simulink model "P702_NI_SoftECU"  (R2019a)
settings: Solver=ode1  StartTime=0.0  StopTime=Inf  FixedStep=0.001  RelTol=1e-3  EnableMultiTasking=on
PreLoadFcn:
  | run '.\VeriStand_BlockSet\NIVeriStandAddPaths.m'
undefined symbols (not defined in the file or in its folder): magnitude
libraries: simulink x83, simulink_extras x1
(part 66 of 76)

== system P702_NI_SoftECU/Output/Subsystem1/To_NI_HIL/Soft_ABS/ABS_BrkBst_Data ==
  in_port : Inport
  BrkTotTqRqDrv_No_Cnt : Terminator
  BrkTotTqRqDrv_No_Cs : Terminator
  BrkTot_Tq_RqDrv : Terminator
  bus_selector : BusSelector  OutputSignals=BrkTot_Tq_RqDrv,BrkTotTqRqDrv_No_Cs,BrkTotTqRqDrv_No_Cnt
  wires:
  in_port/1 -> bus_selector/1  "Subsystem1"
  bus_selector/1 -> BrkTot_Tq_RqDrv/1  "<BrkTot_Tq_RqDrv>"
  bus_selector/2 -> BrkTotTqRqDrv_No_Cs/1  "<BrkTotTqRqDrv_No_Cs>"
  bus_selector/3 -> BrkTotTqRqDrv_No_Cnt/1  "<BrkTotTqRqDrv_No_Cnt>"

== system P702_NI_SoftECU/Output/Subsystem1/To_NI_HIL/Soft_ABS/Accel_Data ==
  in_port : Inport
  VehLat2_A_Actl : Terminator
  VehLong2_A_Actl : Terminator
  bus_selector : BusSelector  OutputSignals=VehLong2_A_Actl,VehLat2_A_Actl
  wires:
  in_port/1 -> bus_selector/1  "Subsystem1"
  bus_selector/1 -> VehLong2_A_Actl/1  "<VehLong2_A_Actl>"
  bus_selector/2 -> VehLat2_A_Actl/1  "<VehLat2_A_Actl>"

== system P702_NI_SoftECU/Output/Subsystem1/To_NI_HIL/Soft_ABS/BrakeSnData_3 ==
  in_port : Inport
  VehLatComp_A_Actl : Terminator
  VehLongComp_A_Actl : Terminator
  VehOverGnd_V_Est : Terminator
  VehYawComp_W_Actl : Terminator
  bus_selector : BusSelector  OutputSignals=VehYawComp_W_Actl,VehOverGnd_V_Est,VehLongComp_A_Actl,VehLatComp_A_Actl
  wires:
  in_port/1 -> bus_selector/1  "Subsystem1"
  bus_selector/1 -> VehYawComp_W_Actl/1  "<VehYawComp_W_Actl>"
  bus_selector/2 -> VehOverGnd_V_Est/1  "<VehOverGnd_V_Est>"
  bus_selector/3 -> VehLongComp_A_Actl/1  "<VehLongComp_A_Actl>"
  bus_selector/4 -> VehLatComp_A_Actl/1  "<VehLatComp_A_Actl>"

== system P702_NI_SoftECU/Output/Subsystem1/To_NI_HIL/Soft_ABS/BrakeSnData_4 ==
  in_port : Inport
  BrkTot_Tq_Actl : Terminator
  VehRolComp_W_Actl : Terminator
  VehVertComp_A_Actl : Terminator
  bus_selector : BusSelector  OutputSignals=VehVertComp_A_Actl,VehRolComp_W_Actl,BrkTot_Tq_Actl
  wires:
  in_port/1 -> bus_selector/1  "Subsystem1"
  bus_selector/1 -> VehVertComp_A_Actl/1  "<VehVertComp_A_Actl>"
  bus_selector/2 -> VehRolComp_W_Actl/1  "<VehRolComp_W_Actl>"
  bus_selector/3 -> BrkTot_Tq_Actl/1  "<BrkTot_Tq_Actl>"

== system P702_NI_SoftECU/Output/Subsystem1/To_NI_HIL/Soft_ABS/BrakeSnData_5 ==
  in_port : Inport
  SteWhlComp_An_Est : Terminator
  bus_selector : BusSelector  OutputSignals=SteWhlComp_An_Est
  wires:
  in_port/1 -> bus_selector/1  "Subsystem1"
  bus_selector/1 -> SteWhlComp_An_Est/1  "<SteWhlComp_An_Est>"

== system P702_NI_SoftECU/Output/Subsystem1/To_NI_HIL/Soft_ABS/BrakeSysFeatures ==
  in_port : Inport
  VehVActlBrk_No_Cnt : Terminator
  VehVActlBrk_No_Cs : Terminator
  Veh_V_ActlBrk : Terminator
  bus_selector : BusSelector  OutputSignals=Veh_V_ActlBrk,VehVActlBrk_No_Cs,VehVActlBrk_No_Cnt
  wires:
  in_port/1 -> bus_selector/1  "Subsystem1"
  bus_selector/1 -> Veh_V_ActlBrk/1  "<Veh_V_ActlBrk>"
  bus_selector/2 -> VehVActlBrk_No_Cs/1  "<VehVActlBrk_No_Cs>"
  bus_selector/3 -> VehVActlBrk_No_Cnt/1  "<VehVActlBrk_No_Cnt>"

== system P702_NI_SoftECU/Output/Subsystem1/To_NI_HIL/Soft_ABS/BrakeSysFeatures_2 ==
  in_port : Inport
  BpedMove_D_Actl : Terminator
  BpedMove_No_Cnt : Terminator
  BpedMove_No_Cs : Terminator
  bus_selector : BusSelector  OutputSignals=BpedMove_D_Actl,BpedMove_No_Cs,BpedMove_No_Cnt
  wires:
  in_port/1 -> bus_selector/1  "Subsystem1"
  bus_selector/1 -> BpedMove_D_Actl/1  "<BpedMove_D_Actl>"
  bus_selector/2 -> BpedMove_No_Cs/1  "<BpedMove_No_Cs>"
  bus_selector/3 -> BpedMove_No_Cnt/1  "<BpedMove_No_Cnt>"

== system P702_NI_SoftECU/Output/Subsystem1/To_NI_HIL/Soft_ABS/DesiredTorqBrk ==
  in_port : Inport
  AccBrkActv_B_Actl : Terminator
  AccBrkPrchgActv_B_Actl : Terminator
  AccBrkTotTqMn_B_Actl : Terminator
  AccStopActv_B_ActlBrk : Terminator
  CmbbBaSensInc_B_Actl : Terminator
  CmbbBrkDecel_B_Actl : Terminator
  CmbbBrkPrchg_B_Actl : Terminator
  VehLongOvrGnd_A_Est : Terminator
  VehStop_D_Stat : Terminator
  VehicleStationary : Terminator
  bus_selector : BusSelector  OutputSignals=AccBrkPrchgActv_B_Actl,AccBrkActv_B_Actl,AccStopActv_B_ActlBrk,CmbbBrkPrchg_B_Actl,CmbbBaSensInc_B_Actl,CmbbBrkDecel_B_Actl,VehicleStationary,VehStop_D_Stat,VehLongOvrGnd_A_Est,AccBrkTotTqMn_B_Actl
  wires:
  in_port/1 -> bus_selector/1  "Subsystem1"
  bus_selector/1 -> AccBrkPrchgActv_B_Actl/1  "<AccBrkPrchgActv_B_Actl>"
  bus_selector/2 -> AccBrkActv_B_Actl/1  "<AccBrkActv_B_Actl>"
  bus_selector/3 -> AccStopActv_B_ActlBrk/1  "<AccStopActv_B_ActlBrk>"
  bus_selector/4 -> CmbbBrkPrchg_B_Actl/1  "<CmbbBrkPrchg_B_Actl>"
  bus_selector/5 -> CmbbBaSensInc_B_Actl/1  "<CmbbBaSensInc_B_Actl>"
  bus_selector/6 -> CmbbBrkDecel_B_Actl/1  "<CmbbBrkDecel_B_Actl>"
  bus_selector/7 -> VehicleStationary/1  "<VehicleStationary>"
  bus_selector/8 -> VehStop_D_Stat/1  "<VehStop_D_Stat>"
  bus_selector/9 -> VehLongOvrGnd_A_Est/1  "<VehLongOvrGnd_A_Est>"
  bus_selector/10 -> AccBrkTotTqMn_B_Actl/1  "<AccBrkTotTqMn_B_Actl>"

== system P702_NI_SoftECU/Output/Subsystem1/To_NI_HIL/Soft_ABS/ToCarSim ==
  in_port : Inport
  MCPressure : Terminator
  bus_selector : BusSelector  OutputSignals=MCPressure
  wires:
  in_port/1 -> bus_selector/1  "Subsystem1"
  bus_selector/1 -> MCPressure/1  "<MCPressure>"

== system P702_NI_SoftECU/Output/Subsystem1/To_NI_HIL/Soft_ABS/WheelData ==
  in_port : Inport
  WhlDirRl_D_Actl : Terminator
  WhlDirRr_D_Actl : Terminator
  bus_selector : BusSelector  OutputSignals=WhlDirRl_D_Actl,WhlDirRr_D_Actl
  wires:
  in_port/1 -> bus_selector/1  "Subsystem1"
  bus_selector/1 -> WhlDirRl_D_Actl/1  "<WhlDirRl_D_Actl>"
  bus_selector/2 -> WhlDirRr_D_Actl/1  "<WhlDirRr_D_Actl>"

== system P702_NI_SoftECU/Output/Subsystem1/To_NI_HIL/Soft_ABS/WheelSpeed ==
  in_port : Inport
  WhlFl_W_Meas : Terminator
  WhlFr_W_Meas : Terminator
  WhlRl_W_Meas : Terminator
  WhlRotatFl_No_Cnt : Terminator
  WhlRotatFr_No_Cnt : Terminator
  WhlRotatRl_No_Cnt : Terminator
  WhlRotatRr_No_Cnt : Terminator
  WhlRr_W_Meas : Terminator
  bus_selector : BusSelector  OutputSignals=WhlFl_W_Meas,WhlFr_W_Meas,WhlRl_W_Meas,WhlRr_W_Meas,WhlRotatFl_No_Cnt,WhlRotatFr_No_Cnt,WhlRotatRl_No_Cnt,WhlRotatRr_No_Cnt
  wires:
  in_port/1 -> bus_selector/1  "Subsystem1"
  bus_selector/1 -> WhlFl_W_Meas/1  "<WhlFl_W_Meas>"
  bus_selector/2 -> WhlFr_W_Meas/1  "<WhlFr_W_Meas>"
  bus_selector/3 -> WhlRl_W_Meas/1  "<WhlRl_W_Meas>"
  bus_selector/4 -> WhlRr_W_Meas/1  "<WhlRr_W_Meas>"
  bus_selector/5 -> WhlRotatFl_No_Cnt/1  "<WhlRotatFl_No_Cnt>"
  bus_selector/6 -> WhlRotatFr_No_Cnt/1  "<WhlRotatFr_No_Cnt>"
  bus_selector/7 -> WhlRotatRl_No_Cnt/1  "<WhlRotatRl_No_Cnt>"
  bus_selector/8 -> WhlRotatRr_No_Cnt/1  "<WhlRotatRr_No_Cnt>"

== system P702_NI_SoftECU/Output/Subsystem1/To_NI_HIL/Soft_ABS/Yaw_Data ==
  in_port : Inport
  VehYaw_W_Actl : Terminator
  bus_selector : BusSelector  OutputSignals=VehYaw_W_Actl
  wires:
  in_port/1 -> bus_selector/1  "Subsystem1"
  bus_selector/1 -> VehYaw_W_Actl/1  "<VehYaw_W_Actl>"

== system P702_NI_SoftECU/Output/Subsystem1/To_NI_HIL/Soft_BCM/BodyInfo_3 ==
  in_port : Inport
  Ignition_Status : Terminator
  bus_selector : BusSelector  OutputSignals=Ignition_Status
  wires:
  in_port/1 -> bus_selector/1  "Subsystem1"
  bus_selector/1 -> Ignition_Status/1  "<Ignition_Status>"

== system P702_NI_SoftECU/Output/Subsystem1/To_NI_HIL/Soft_BCM/Cluster_Info1 ==
  in_port : Inport
  OdometerMasterValue : Terminator
  OdometerMasterValue_UB : Terminator
  bus_selector : BusSelector  OutputSignals=OdometerMasterValue,OdometerMasterValue_UB
  wires:
  in_port/1 -> bus_selector/1  "Subsystem1"
  bus_selector/1 -> OdometerMasterValue/1  "<OdometerMasterValue>"
  bus_selector/2 -> OdometerMasterValue_UB/1  "<OdometerMasterValue_UB>"

== system P702_NI_SoftECU/Output/Subsystem1/To_NI_HIL/Soft_BCM/GGCC_Config_Mgmt_ID ==
  in_port : Inport
  Byte_{0..7} (8 alike) : Terminator
  bus_selector : BusSelector  OutputSignals=Byte_0,Byte_1,Byte_2,Byte_3,Byte_4,Byte_5,Byte_6,Byte_7
  wires:
  in_port/1 -> bus_selector/1  "Subsystem1"
  bus_selector/1 -> Byte_0/1  "<Byte_0>"
  bus_selector/2 -> Byte_1/1  "<Byte_1>"
  bus_selector/3 -> Byte_2/1  "<Byte_2>"
  bus_selector/4 -> Byte_3/1  "<Byte_3>"
  bus_selector/5 -> Byte_4/1  "<Byte_4>"
  bus_selector/6 -> Byte_5/1  "<Byte_5>"
  bus_selector/7 -> Byte_6/1  "<Byte_6>"
  bus_selector/8 -> Byte_7/1  "<Byte_7>"

== system P702_NI_SoftECU/Output/Subsystem1/To_NI_HIL/Soft_BCM/Personality_BCM2_Data ==
  in_port : Inport
  RecallEvent_No_Cnt : Terminator
  bus_selector : BusSelector  OutputSignals=RecallEvent_No_Cnt
  wires:
  in_port/1 -> bus_selector/1  "Subsystem1"
  bus_selector/1 -> RecallEvent_No_Cnt/1  "<RecallEvent_No_Cnt>"

== system P702_NI_SoftECU/Output/Subsystem1/To_NI_HIL/Soft_ECM/EngBrakeData ==
  in_port : Inport
  ACCStopMde_D_Rq : Terminator
  Cc_Stat_D_Actl : Terminator
  CmbbEngTqMn_B_Rq : Terminator
  PrplTqMnSat_B_Actl : Terminator
  bus_selector : BusSelector  OutputSignals=CmbbEngTqMn_B_Rq,ACCStopMde_D_Rq,PrplTqMnSat_B_Actl,Cc_Stat_D_Actl
  wires:
  in_port/1 -> bus_selector/1  "Subsystem1"
  bus_selector/1 -> CmbbEngTqMn_B_Rq/1  "<CmbbEngTqMn_B_Rq>"
  bus_selector/2 -> ACCStopMde_D_Rq/1  "<ACCStopMde_D_Rq>"
  bus_selector/3 -> PrplTqMnSat_B_Actl/1  "<PrplTqMnSat_B_Actl>"
  bus_selector/4 -> Cc_Stat_D_Actl/1  "<Cc_Stat_D_Actl>"

== system P702_NI_SoftECU/Output/Subsystem1/To_NI_HIL/Soft_ECM/EngVehicleSpThrottle ==
  in_port : Inport
  EngAout_N_Actl : Terminator
  bus_selector : BusSelector  OutputSignals=EngAout_N_Actl
  wires:
  in_port/1 -> bus_selector/1  "Subsystem1"
  bus_selector/1 -> EngAout_N_Actl/1  "<EngAout_N_Actl>"

== system P702_NI_SoftECU/Output/Subsystem1/To_NI_HIL/Soft_ECM/EngVehicleSpThrottle2 ==
  in_port : Inport
  Veh_V_ActlEng : Terminator
  bus_selector : BusSelector  OutputSignals=Veh_V_ActlEng
  wires:
  in_port/1 -> bus_selector/1  "Subsystem1"
  bus_selector/1 -> Veh_V_ActlEng/1  "<Veh_V_ActlEng>"

== system P702_NI_SoftECU/Output/Subsystem1/To_NI_HIL/Soft_MRR/MRR_Detection ==
  in_port : Inport
  MRR_Detection_001 : Subsystem
  MRR_Detection_002 : Subsystem
  MRR_Detection_003 : Subsystem
  bus_selector : BusSelector  OutputSignals=MRR_Detection_001,MRR_Detection_002,MRR_Detection_003
  wires:
  in_port/1 -> bus_selector/1  "Subsystem1"
  bus_selector/1 -> MRR_Detection_001/1(in_port)  "<MRR_Detection_001>"
  bus_selector/2 -> MRR_Detection_002/1(in_port)  "<MRR_Detection_002>"
  bus_selector/3 -> MRR_Detection_003/1(in_port)  "<MRR_Detection_003>"

== system P702_NI_SoftECU/Output/Subsystem1/To_NI_HIL/Soft_PCM/EngBrakeData ==
  in_port : Inport
  BpedDrvAppl_D_Actl : Terminator
  BrkOnOffSwtch_D_Actl : Terminator
  bus_selector : BusSelector  OutputSignals=BrkOnOffSwtch_D_Actl,BpedDrvAppl_D_Actl
  wires:
  in_port/1 -> bus_selector/1  "Subsystem1"
  bus_selector/1 -> BrkOnOffSwtch_D_Actl/1  "<BrkOnOffSwtch_D_Actl>"
  bus_selector/2 -> BpedDrvAppl_D_Actl/1  "<BpedDrvAppl_D_Actl>"

== system P702_NI_SoftECU/Output/Subsystem1/To_NI_HIL/Soft_PCM/EngVehicleSpThottle2 ==
  in_port : Inport
  GearRvrse_D_Actl : Terminator
  Veh_V_ActlEng : Terminator
  Veh_V_RqCcSet : Terminator
  bus_selector : BusSelector  OutputSignals=Veh_V_ActlEng,GearRvrse_D_Actl,Veh_V_RqCcSet
  wires:
  in_port/1 -> bus_selector/1  "Subsystem1"
  bus_selector/1 -> Veh_V_ActlEng/1  "<Veh_V_ActlEng>"
  bus_selector/2 -> GearRvrse_D_Actl/1  "<GearRvrse_D_Actl>"
  bus_selector/3 -> Veh_V_RqCcSet/1  "<Veh_V_RqCcSet>"

== system P702_NI_SoftECU/Output/Subsystem1/To_NI_HIL/Soft_PCM/EngVehicleSpThrottle ==
  in_port : Inport
  ApedPosPcActl_No_Cs : Terminator
  ApedPos_PcRate_ActlArb : Terminator
  ApedPos_Pc_ActlArb : Terminator
  ApedPos_Pc_ActlArb_No_Cnt : Terminator
  EngAout_N_Actl : Terminator
  bus_selector : BusSelector  OutputSignals=EngAout_N_Actl,ApedPos_Pc_ActlArb,ApedPos_PcRate_ActlArb,ApedPosPcActl_No_Cs,ApedPos_Pc_ActlArb_No_Cnt
  wires:
  in_port/1 -> bus_selector/1  "Subsystem1"
  bus_selector/1 -> EngAout_N_Actl/1  "<EngAout_N_Actl>"
  bus_selector/2 -> ApedPos_Pc_ActlArb/1  "<ApedPos_Pc_ActlArb>"
  bus_selector/3 -> ApedPos_PcRate_ActlArb/1  "<ApedPos_PcRate_ActlArb>"
  bus_selector/4 -> ApedPosPcActl_No_Cs/1  "<ApedPosPcActl_No_Cs>"
  bus_selector/5 -> ApedPos_Pc_ActlArb_No_Cnt/1  "<ApedPos_Pc_ActlArb_No_Cnt>"

== system P702_NI_SoftECU/Output/Subsystem1/To_NI_HIL/Soft_PCM/EngineClimateData ==
  in_port : Inport
  AirAmb_Te_Actl : Terminator
  AirAmb_Te_ActlFilt : Terminator
  EngAout_Aa_Actl : Terminator
  bus_selector : BusSelector  OutputSignals=EngAout_Aa_Actl,AirAmb_Te_Actl,AirAmb_Te_ActlFilt
  wires:
  in_port/1 -> bus_selector/1  "Subsystem1"
  bus_selector/1 -> EngAout_Aa_Actl/1  "<EngAout_Aa_Actl>"
  bus_selector/2 -> AirAmb_Te_Actl/1  "<AirAmb_Te_Actl>"
  bus_selector/3 -> AirAmb_Te_ActlFilt/1  "<AirAmb_Te_ActlFilt>"

== system P702_NI_SoftECU/Output/Subsystem1/To_NI_HIL/Soft_PCM/EngineClutchData ==
  in_port : Inport
  CluPdlPosPcMeas_D_Qf : Terminator
  CluPdlPos_Pc_Meas : Terminator
  CluPdl_PcRate_Actl : Terminator
  bus_selector : BusSelector  OutputSignals=CluPdl_PcRate_Actl,CluPdlPos_Pc_Meas,CluPdlPosPcMeas_D_Qf
  wires:
  in_port/1 -> bus_selector/1  "Subsystem1"
  bus_selector/1 -> CluPdl_PcRate_Actl/1  "<CluPdl_PcRate_Actl>"
  bus_selector/2 -> CluPdlPos_Pc_Meas/1  "<CluPdlPos_Pc_Meas>"
  bus_selector/3 -> CluPdlPosPcMeas_D_Qf/1  "<CluPdlPosPcMeas_D_Qf>"

== system P702_NI_SoftECU/Output/Subsystem1/To_NI_HIL/Soft_PCM/EngineData_7 ==
  in_port : Inport
  FuelFlw_Vl_Dsply : Terminator
  OdoCount : Terminator
  bus_selector : BusSelector  OutputSignals=OdoCount,FuelFlw_Vl_Dsply
  wires:
  in_port/1 -> bus_selector/1  "Subsystem1"
  bus_selector/1 -> OdoCount/1  "<OdoCount>"
  bus_selector/2 -> FuelFlw_Vl_Dsply/1  "<FuelFlw_Vl_Dsply>"

== system P702_NI_SoftECU/Output/Subsystem1/To_NI_HIL/Soft_PCM/PowertrainData_10 ==
  in_port : Inport
  GearLvr_D_ActlDrv : Terminator
  GearPos_No_Cnt : Terminator
  GearPos_No_Cs : Terminator
  bus_selector : BusSelector  OutputSignals=GearPos_No_Cs,GearPos_No_Cnt,GearLvr_D_ActlDrv
  wires:
  in_port/1 -> bus_selector/1  "Subsystem1"
  bus_selector/1 -> GearPos_No_Cs/1  "<GearPos_No_Cs>"
  bus_selector/2 -> GearPos_No_Cnt/1  "<GearPos_No_Cnt>"
  bus_selector/3 -> GearLvr_D_ActlDrv/1  "<GearLvr_D_ActlDrv>"

== system P702_NI_SoftECU/Output/Subsystem1/To_NI_HIL/Soft_PCM/TorqueDataEngFlags ==
  in_port : Inport
  PrplWhlTotTqRq_No_Cs : Terminator
  PrplWhlTot_Tq_Rq : Terminator
  PrplWhlTot_Tq_Rq_No_Cnt : Terminator
  bus_selector : BusSelector  OutputSignals=PrplWhlTot_Tq_Rq,PrplWhlTotTqRq_No_Cs,PrplWhlTot_Tq_Rq_No_Cnt
  wires:
  in_port/1 -> bus_selector/1  "Subsystem1"
  bus_selector/1 -> PrplWhlTot_Tq_Rq/1  "<PrplWhlTot_Tq_Rq>"
  bus_selector/2 -> PrplWhlTotTqRq_No_Cs/1  "<PrplWhlTotTqRq_No_Cs>"
  bus_selector/3 -> PrplWhlTot_Tq_Rq_No_Cnt/1  "<PrplWhlTot_Tq_Rq_No_Cnt>"

== system P702_NI_SoftECU/Output/Subsystem1/To_NI_HIL/Soft_PCM/VehicleOperatingModes ==
  in_port : Inport
  ElPw_D_Stat : Terminator
  ElPw_D_StatStrtStop : Terminator
  Eng_D_Stat : Terminator
  PrplWhlTot2_Tq_Rq : Terminator
  PwPckTq_D_Stat : Terminator
  bus_selector : BusSelector  OutputSignals=Eng_D_Stat,PwPckTq_D_Stat,PrplWhlTot2_Tq_Rq,ElPw_D_StatStrtStop,ElPw_D_Stat
  wires:
  in_port/1 -> bus_selector/1  "Subsystem1"
  bus_selector/1 -> Eng_D_Stat/1  "<Eng_D_Stat>"
  bus_selector/2 -> PwPckTq_D_Stat/1  "<PwPckTq_D_Stat>"
  bus_selector/3 -> PrplWhlTot2_Tq_Rq/1  "<PrplWhlTot2_Tq_Rq>"
  bus_selector/4 -> ElPw_D_StatStrtStop/1  "<ElPw_D_StatStrtStop>"
  bus_selector/5 -> ElPw_D_Stat/1  "<ElPw_D_Stat>"

== system P702_NI_SoftECU/Output/Subsystem1/To_NI_HIL/Soft_RCM/Accel_Data ==
  in_port : Inport
  VehLat2_A_Actl : Terminator
  VehLatAActl_D_Qf : Terminator
  VehLatLongVert_No_Cnt : Terminator
  VehLatLongVert_No_Cs : Terminator
  VehLong2_A_Actl : Terminator
  VehLongAActl_D_Qf : Terminator
  VehVert2_A_Actl : Terminator
  VehVertAActl_D_Qf : Terminator
  bus_selector : BusSelector  OutputSignals=VehLat2_A_Actl,VehLong2_A_Actl,VehVert2_A_Actl,VehLatLongVert_No_Cnt,VehLatLongVert_No_Cs,VehLatAActl_D_Qf,VehLongAActl_D_Qf,VehVertAActl_D_Qf
  wires:
  in_port/1 -> bus_selector/1  "Subsystem1"
  bus_selector/1 -> VehLat2_A_Actl/1  "<VehLat2_A_Actl>"
  bus_selector/2 -> VehLong2_A_Actl/1  "<VehLong2_A_Actl>"
  bus_selector/3 -> VehVert2_A_Actl/1  "<VehVert2_A_Actl>"
  bus_selector/4 -> VehLatLongVert_No_Cnt/1  "<VehLatLongVert_No_Cnt>"
  bus_selector/5 -> VehLatLongVert_No_Cs/1  "<VehLatLongVert_No_Cs>"
  bus_selector/6 -> VehLatAActl_D_Qf/1  "<VehLatAActl_D_Qf>"
  bus_selector/7 -> VehLongAActl_D_Qf/1  "<VehLongAActl_D_Qf>"
  bus_selector/8 -> VehVertAActl_D_Qf/1  "<VehVertAActl_D_Qf>"

== system P702_NI_SoftECU/Output/Subsystem1/To_NI_HIL/Soft_RCM/RCMStatusMessage2 ==
  in_port : Inport
  FirstRowBuckleDriver : Terminator
  RstrnImpactEvntStatus : Terminator
  bus_selector : BusSelector  OutputSignals=RstrnImpactEvntStatus,FirstRowBuckleDriver
  wires:
  in_port/1 -> bus_selector/1  "Subsystem1"
  bus_selector/1 -> RstrnImpactEvntStatus/1  "<RstrnImpactEvntStatus>"
  bus_selector/2 -> FirstRowBuckleDriver/1  "<FirstRowBuckleDriver>"

== system P702_NI_SoftECU/Output/Subsystem1/To_NI_HIL/Soft_RCM/Yaw_Data ==
  in_port : Inport
  VehRolWActl_D_Qf : Terminator
  VehRol_W_Actl : Terminator
  VehRollYawW_No_Cs : Terminator
  VehRollYaw_No_Cnt : Terminator
  VehYawWActl_D_Qf : Terminator
  VehYaw_W_Actl : Terminator
  bus_selector : BusSelector  OutputSignals=VehRol_W_Actl,VehYaw_W_Actl,VehRollYaw_No_Cnt,VehRollYawW_No_Cs,VehRolWActl_D_Qf,VehYawWActl_D_Qf
  wires:
  in_port/1 -> bus_selector/1  "Subsystem1"
  bus_selector/1 -> VehRol_W_Actl/1  "<VehRol_W_Actl>"
  bus_selector/2 -> VehYaw_W_Actl/1  "<VehYaw_W_Actl>"
  bus_selector/3 -> VehRollYaw_No_Cnt/1  "<VehRollYaw_No_Cnt>"
  bus_selector/4 -> VehRollYawW_No_Cs/1  "<VehRollYawW_No_Cs>"
  bus_selector/5 -> VehRolWActl_D_Qf/1  "<VehRolWActl_D_Qf>"
  bus_selector/6 -> VehYawWActl_D_Qf/1  "<VehYawWActl_D_Qf>"

== system P702_NI_SoftECU/Output/Subsystem1/To_NI_HIL/Soft_SCCM/Steering_Data ==
  in_port : Inport
  AccButtnGapDecPress : Terminator
  AccButtnGapIncPress : Terminator
  AhbStat_B_Dsply : Terminator
  AslButtnOnOffCnclPress : Terminator
  AslButtnOnOffPress : Terminator
  CcAslButtnCnclPress : Terminator
  CcAslButtnCnclResPress : Terminator
  CcAslButtnOnPress : Terminator
  CcAslButtnResDecPress : Terminator
  CcAslButtnResIncPress : Terminator
  CcAslButtnSetDecPress : Terminator
  CcAslButtnSetIncPress : Terminator
  CcAslButtnSetPress : Terminator
  CcAsllButtnResPress : Terminator
  CcButtnOffPress : Terminator
  CcButtnOnOffCnclPress : Terminator
  CcButtnOnOffPress : Terminator
  CcButtnOnPress : Terminator
  HeadLghtHiCtrl_D_RqAhb : Terminator
  HeadLghtHiOn_B_StatAhb : Terminator
  bus_selector : BusSelector  OutputSignals=AhbStat_B_Dsply,HeadLghtHiCtrl_D_RqAhb,HeadLghtHiOn_B_StatAhb,CcButtnOnPress,CcButtnOffPress,CcAslButtnCnclPress,CcAsllButtnResPress,CcAslButtnResIncPress,CcAslButtnSetIncPress,CcAslButtnSetDecPress,CcAslButtnSetPress,AccButtnGapIncPress,AccButtnGapDecPress,AslButtnOnOffPress,AslButtnOnOffCnclPress,CcButtnOnOffPress,CcButtnOnOffCnclPress,CcAslButtnResDecPress,CcAslButtnOnPress,CcAslButtnCnclResPress
  wires:
  in_port/1 -> bus_selector/1  "Subsystem1"
  bus_selector/1 -> AhbStat_B_Dsply/1  "<AhbStat_B_Dsply>"
  bus_selector/2 -> HeadLghtHiCtrl_D_RqAhb/1  "<HeadLghtHiCtrl_D_RqAhb>"
  bus_selector/3 -> HeadLghtHiOn_B_StatAhb/1  "<HeadLghtHiOn_B_StatAhb>"
  bus_selector/4 -> CcButtnOnPress/1  "<CcButtnOnPress>"
  bus_selector/5 -> CcButtnOffPress/1  "<CcButtnOffPress>"
  bus_selector/6 -> CcAslButtnCnclPress/1  "<CcAslButtnCnclPress>"
  bus_selector/7 -> CcAsllButtnResPress/1  "<CcAsllButtnResPress>"
  bus_selector/8 -> CcAslButtnResIncPress/1  "<CcAslButtnResIncPress>"
  bus_selector/9 -> CcAslButtnSetIncPress/1  "<CcAslButtnSetIncPress>"
  bus_selector/10 -> CcAslButtnSetDecPress/1  "<CcAslButtnSetDecPress>"
  bus_selector/11 -> CcAslButtnSetPress/1  "<CcAslButtnSetPress>"
  bus_selector/12 -> AccButtnGapIncPress/1  "<AccButtnGapIncPress>"
  bus_selector/13 -> AccButtnGapDecPress/1  "<AccButtnGapDecPress>"
  bus_selector/14 -> AslButtnOnOffPress/1  "<AslButtnOnOffPress>"
  bus_selector/15 -> AslButtnOnOffCnclPress/1  "<AslButtnOnOffCnclPress>"
  bus_selector/16 -> CcButtnOnOffPress/1  "<CcButtnOnOffPress>"
  bus_selector/17 -> CcButtnOnOffCnclPress/1  "<CcButtnOnOffCnclPress>"
  bus_selector/18 -> CcAslButtnResDecPress/1  "<CcAslButtnResDecPress>"
  bus_selector/19 -> CcAslButtnOnPress/1  "<CcAslButtnOnPress>"
  bus_selector/20 -> CcAslButtnCnclResPress/1  "<CcAslButtnCnclResPress>"

== system P702_NI_SoftECU/Output/Subsystem1/To_NI_HIL/Soft_SCCM/Steering_Wheel_Data2 ==
  in_port : Inport
  SteWhlSwtchBack_B_Stat : Terminator
  SteWhlSwtchDown_B_Stat : Terminator
  SteWhlSwtchLeft_B_Stat : Terminator
  SteWhlSwtchMenu_B_Stat : Terminator
  SteWhlSwtchOk_B_Stat : Terminator
  SteWhlSwtchRght_B_Stat : Terminator
  SteWhlSwtchUp_B_Stat : Terminator
  bus_selector : BusSelector  OutputSignals=SteWhlSwtchOk_B_Stat,SteWhlSwtchUp_B_Stat,SteWhlSwtchDown_B_Stat,SteWhlSwtchLeft_B_Stat,SteWhlSwtchRght_B_Stat,SteWhlSwtchMenu_B_Stat,SteWhlSwtchBack_B_Stat
  wires:
  in_port/1 -> bus_selector/1  "Subsystem1"
  bus_selector/1 -> SteWhlSwtchOk_B_Stat/1  "<SteWhlSwtchOk_B_Stat>"
  bus_selector/2 -> SteWhlSwtchUp_B_Stat/1  "<SteWhlSwtchUp_B_Stat>"
  bus_selector/3 -> SteWhlSwtchDown_B_Stat/1  "<SteWhlSwtchDown_B_Stat>"
  bus_selector/4 -> SteWhlSwtchLeft_B_Stat/1  "<SteWhlSwtchLeft_B_Stat>"
  bus_selector/5 -> SteWhlSwtchRght_B_Stat/1  "<SteWhlSwtchRght_B_Stat>"
  bus_selector/6 -> SteWhlSwtchMenu_B_Stat/1  "<SteWhlSwtchMenu_B_Stat>"
  bus_selector/7 -> SteWhlSwtchBack_B_Stat/1  "<SteWhlSwtchBack_B_Stat>"

== system P702_NI_SoftECU/Output/Subsystem1/To_NI_HIL/Soft_TCM/TransGearData ==
  in_port : Inport
  GearLvrPos_D_Actl : Terminator
  bus_selector : BusSelector  OutputSignals=GearLvrPos_D_Actl
  wires:
  in_port/1 -> bus_selector/1  "Subsystem1"
  bus_selector/1 -> GearLvrPos_D_Actl/1  "<GearLvrPos_D_Actl>"

== system P702_NI_SoftECU/Output/Subsystem2/CAN_Signal/ABS_ESC/ABS_AutoSar_NetworkMgt_0x596 ==
  ABS_AutoSarNMControl : Constant  Value=0
  ABS_AutoSarNMNodeId : Constant  Value=0
  ABS_AutoSarNMReserved{1..4} (4 alike) : Constant  Value=0
  ABS_GWNMProxy : Constant  Value=0
  ABS_GWOnBoardTester : Constant  Value=0
  bus_creator : BusCreator  Inputs=8
  out_port : Outport
  wires:
  bus_creator/1 -> out_port/1  "Subsystem2"
  ABS_AutoSarNMNodeId/1 -> bus_creator/1  "ABS_AutoSarNMNodeId"
  ABS_AutoSarNMControl/1 -> bus_creator/2  "ABS_AutoSarNMControl"
  ABS_AutoSarNMReserved1/1 -> bus_creator/3  "ABS_AutoSarNMReserved1"
  ABS_AutoSarNMReserved2/1 -> bus_creator/4  "ABS_AutoSarNMReserved2"
  ABS_GWOnBoardTester/1 -> bus_creator/5  "ABS_GWOnBoardTester"
  ABS_GWNMProxy/1 -> bus_creator/6  "ABS_GWNMProxy"
  ABS_AutoSarNMReserved3/1 -> bus_creator/7  "ABS_AutoSarNMReserved3"
  ABS_AutoSarNMReserved4/1 -> bus_creator/8  "ABS_AutoSarNMReserved4"

== system P702_NI_SoftECU/Output/Subsystem2/CAN_Signal/ABS_ESC/ABS_BrkBst_Data_0x4B0 ==
  BrkAutoHold_D_Stat : Constant  Value=0
  BrkBstrVac_P_Actl : Constant  Value=0
  BrkTotTqRqDrv_No_Cnt : Constant  Value=0
  BrkTotTqRqDrv_No_Cs : Constant  Value=0
  BrkTot_Tq_RqDrv : Constant  Value=0
  HsaStat_D_Dsply : Constant  Value=0
  HsaTrnAout_Tq_Rq : Constant  Value=0
  YawStabilityIndex : Constant  Value=0
  bus_creator : BusCreator  Inputs=8
  out_port : Outport
  wires:
  bus_creator/1 -> out_port/1  "Subsystem2"
  BrkBstrVac_P_Actl/1 -> bus_creator/1  "BrkBstrVac_P_Actl"
  YawStabilityIndex/1 -> bus_creator/2  "YawStabilityIndex"
  HsaTrnAout_Tq_Rq/1 -> bus_creator/3  "HsaTrnAout_Tq_Rq"
  BrkTotTqRqDrv_No_Cnt/1 -> bus_creator/4  "BrkTotTqRqDrv_No_Cnt"
  BrkAutoHold_D_Stat/1 -> bus_creator/5  "BrkAutoHold_D_Stat"
  BrkTot_Tq_RqDrv/1 -> bus_creator/6  "BrkTot_Tq_RqDrv"
  HsaStat_D_Dsply/1 -> bus_creator/7  "HsaStat_D_Dsply"
  BrkTotTqRqDrv_No_Cs/1 -> bus_creator/8  "BrkTotTqRqDrv_No_Cs"

== system P702_NI_SoftECU/Output/Subsystem2/CAN_Signal/ABS_ESC/ABS_Rapid_Data_Response_1_0x6B0 ==
  UUDTABSResponse1 : Constant  Value=0
  bus_creator : BusCreator  Inputs=1
  out_port : Outport
  wires:
  bus_creator/1 -> out_port/1  "Subsystem2"
  UUDTABSResponse1/1 -> bus_creator/1  "UUDTABSResponse1"

== system P702_NI_SoftECU/Output/Subsystem2/CAN_Signal/ABS_ESC/ABS_Rapid_Data_Response_2_0x6B1 ==
  UUDTABSResponse2 : Constant  Value=0
  bus_creator : BusCreator  Inputs=1
  out_port : Outport
  wires:
  bus_creator/1 -> out_port/1  "Subsystem2"
  UUDTABSResponse2/1 -> bus_creator/1  "UUDTABSResponse2"

== system P702_NI_SoftECU/Output/Subsystem2/CAN_Signal/ABS_ESC/ActiveFronSteering_Req_0x88 ==
  SteWhlBrkAnRq_No_Cnt : Constant  Value=0
  SteWhlBrkAnRq_No_Cs : Constant  Value=0
  SteWhlBrkOffst_An_Rq : Constant  Value=0
  bus_creator : BusCreator  Inputs=3
  out_port : Outport
  wires:
  bus_creator/1 -> out_port/1  "Subsystem2"
  SteWhlBrkOffst_An_Rq/1 -> bus_creator/1  "SteWhlBrkOffst_An_Rq"
  SteWhlBrkAnRq_No_Cs/1 -> bus_creator/2  "SteWhlBrkAnRq_No_Cs"
  SteWhlBrkAnRq_No_Cnt/1 -> bus_creator/3  "SteWhlBrkAnRq_No_Cnt"

== system P702_NI_SoftECU/Output/Subsystem2/CAN_Signal/ABS_ESC/BrakeSnData_3_0x77 ==
  VehLatComp_A_Actl : Constant  Value=0
  VehLongComp_A_Actl : Constant  Value=0
  VehOverGnd_V_Est : Constant  Value=0
  VehTrvlDir_D_Stat : Constant  Value=0
  VehYawComp_W_Actl : Constant  Value=0
  bus_creator : BusCreator  Inputs=5
  out_port : Outport
  wires:
  bus_creator/1 -> out_port/1  "Subsystem2"
  VehOverGnd_V_Est/1 -> bus_creator/1  "VehOverGnd_V_Est"
  VehTrvlDir_D_Stat/1 -> bus_creator/2  "VehTrvlDir_D_Stat"
  VehYawComp_W_Actl/1 -> bus_creator/3  "VehYawComp_W_Actl"
  VehLatComp_A_Actl/1 -> bus_creator/4  "VehLatComp_A_Actl"
  VehLongComp_A_Actl/1 -> bus_creator/5  "VehLongComp_A_Actl"

== system P702_NI_SoftECU/Output/Subsystem2/CAN_Signal/ABS_ESC/BrakeSnData_4_0x7D ==
  BrkTotTqRqArb_No_Cnt : Constant  Value=0
  BrkTotTqRqArb_No_Cs : Constant  Value=0
  BrkTot_Tq_Actl : Constant  Value=0
  BrkTot_Tq_RqArb : Constant  Value=0
  HsaStat_D_Actl : Constant  Value=0
  VehRolComp_W_Actl : Constant  Value=0
  VehVertComp_A_Actl : Constant  Value=0
  bus_creator : BusCreator  Inputs=7
  out_port : Outport
  wires:
  bus_creator/1 -> out_port/1  "Subsystem2"
  HsaStat_D_Actl/1 -> bus_creator/1  "HsaStat_D_Actl"
  BrkTot_Tq_RqArb/1 -> bus_creator/2  "BrkTot_Tq_RqArb"
  BrkTotTqRqArb_No_Cs/1 -> bus_creator/3  "BrkTotTqRqArb_No_Cs"
  BrkTotTqRqArb_No_Cnt/1 -> bus_creator/4  "BrkTotTqRqArb_No_Cnt"
  BrkTot_Tq_Actl/1 -> bus_creator/5  "BrkTot_Tq_Actl"
  VehVertComp_A_Actl/1 -> bus_creator/6  "VehVertComp_A_Actl"
  VehRolComp_W_Actl/1 -> bus_creator/7  "VehRolComp_W_Actl"

== system P702_NI_SoftECU/Output/Subsystem2/CAN_Signal/ABS_ESC/BrakeSnData_5_0x76 ==
  AwdLck_Tq_RqMn : Constant  Value=0
  AwdLck_Tq_RqMx : Constant  Value=0
  BrkCtrFnd_B_Stat : Constant  Value=0
  DrvSte_D_Stat : Constant  Value=0
  DrvSte_Tq_Rq : Constant  Value=0
  EmgcyBrkLamp_D_Rq : Constant  Value=0
  SteWhlCompAnEst_D_Qf : Constant  Value=0
  SteWhlComp_An_Est : Constant  Value=0
  StopLamp_B_RqBrk : Constant  Value=0
  bus_creator : BusCreator  Inputs=9
  out_port : Outport
  wires:
  bus_creator/1 -> out_port/1  "Subsystem2"
  StopLamp_B_RqBrk/1 -> bus_creator/1  "StopLamp_B_RqBrk"
  SteWhlComp_An_Est/1 -> bus_creator/2  "SteWhlComp_An_Est"
  SteWhlCompAnEst_D_Qf/1 -> bus_creator/3  "SteWhlCompAnEst_D_Qf"
  EmgcyBrkLamp_D_Rq/1 -> bus_creator/4  "EmgcyBrkLamp_D_Rq"
  DrvSte_D_Stat/1 -> bus_creator/5  "DrvSte_D_Stat"
  DrvSte_Tq_Rq/1 -> bus_creator/6  "DrvSte_Tq_Rq"
  BrkCtrFnd_B_Stat/1 -> bus_creator/7  "BrkCtrFnd_B_Stat"
  AwdLck_Tq_RqMx/1 -> bus_creator/8  "AwdLck_Tq_RqMx"
  AwdLck_Tq_RqMn/1 -> bus_creator/9  "AwdLck_Tq_RqMn"

== system P702_NI_SoftECU/Output/Subsystem2/CAN_Signal/ABS_ESC/BrakeSnData_6_0x414 ==
  StePinOffst_An_Est : Constant  Value=0
  StePinOffst_D_Stat : Constant  Value=0
  StePinOffst_No_Cnt : Constant  Value=0
  StePinOffst_No_Cs : Constant  Value=0
  bus_creator : BusCreator  Inputs=4
  out_port : Outport
  wires:
  bus_creator/1 -> out_port/1  "Subsystem2"
  StePinOffst_An_Est/1 -> bus_creator/1  "StePinOffst_An_Est"
  StePinOffst_D_Stat/1 -> bus_creator/2  "StePinOffst_D_Stat"
  StePinOffst_No_Cnt/1 -> bus_creator/3  "StePinOffst_No_Cnt"
  StePinOffst_No_Cs/1 -> bus_creator/4  "StePinOffst_No_Cs"

== system P702_NI_SoftECU/Output/Subsystem2/CAN_Signal/ABS_ESC/BrakeSysFeatures_0x415 ==
  BrkFluidLvl_D_Stat : Constant  Value=0
  LsmcBrkDecel_D_Stat : Constant  Value=0
  VehStab_D_Stat : Constant  Value=0
  VehVActlBrk_D_Qf : Constant  Value=0
  VehVActlBrk_No_Cnt : Constant  Value=0
  VehVActlBrk_No_Cs : Constant  Value=0
  VehYawLin_W_Rq : Constant  Value=0
  VehYawNonLin_W_Rq : Constant  Value=0
  Veh_V_ActlBrk : Constant  Value=0
  bus_creator : BusCreator  Inputs=9
  out_port : Outport
  wires:
  bus_creator/1 -> out_port/1  "Subsystem2"
  Veh_V_ActlBrk/1 -> bus_creator/1  "Veh_V_ActlBrk"
  VehVActlBrk_D_Qf/1 -> bus_creator/2  "VehVActlBrk_D_Qf"
  VehVActlBrk_No_Cnt/1 -> bus_creator/3  "VehVActlBrk_No_Cnt"
  BrkFluidLvl_D_Stat/1 -> bus_creator/4  "BrkFluidLvl_D_Stat"
  VehVActlBrk_No_Cs/1 -> bus_creator/5  "VehVActlBrk_No_Cs"
  LsmcBrkDecel_D_Stat/1 -> bus_creator/6  "LsmcBrkDecel_D_Stat"
  VehYawLin_W_Rq/1 -> bus_creator/7  "VehYawLin_W_Rq"
  VehStab_D_Stat/1 -> bus_creator/8  "VehStab_D_Stat"
  VehYawNonLin_W_Rq/1 -> bus_creator/9  "VehYawNonLin_W_Rq"

== system P702_NI_SoftECU/Output/Subsystem2/CAN_Signal/ABS_ESC/BrakeSysFeatures_2_0x416 ==
  Abs_B_Falt : Constant  Value=0
  BpedMove_D_Actl : Constant  Value=0
  BpedMove_No_Cnt : Constant  Value=0
  BrkBstrVac_B_Rq : Constant  Value=0
  BrkLamp_B_Rq : Constant  Value=0
  ChimeBrk_B_Rq : Constant  Value=0
  DrvAntiLckLamp_D_Rq : Constant  Value=0
  DrvHdcLampInfo_D_Rq : Constant  Value=0
  DrvHdcMsg_D_Rq : Constant  Value=0
  DrvHdcWarnInfo_D_Rq : Constant  Value=0
  DrvSlipCtlLamp_D_Rq : Constant  Value=0
  DrvSlipCtlMde_D_Ind : Constant  Value=0
  HILL_DESC_MC : Constant  Value=0
  HdcMde_D_Actl : Constant  Value=0
  HsaMde_D_Mem : Constant  Value=0
  RearDiffElckrOpen_B_Rq : Constant  Value=0
  RearDiffLck_Tq2_RqMx : Constant  Value=0
  StabCtlBrk_B_Avail : Constant  Value=0
  TCMode : Constant  Value=0
  TRLR_SWAY_CONFIG_STAT : Constant  Value=0
  TRLR_SWAY_EVNT_IN_PROG : Constant  Value=0
  bus_creator : BusCreator  Inputs=21
  out_port : Outport
  wires:
  bus_creator/1 -> out_port/1  "Subsystem2"
  BpedMove_D_Actl/1 -> bus_creator/1  "BpedMove_D_Actl"
  Abs_B_Falt/1 -> bus_creator/2  "Abs_B_Falt"
  StabCtlBrk_B_Avail/1 -> bus_creator/3  "StabCtlBrk_B_Avail"
  BpedMove_No_Cnt/1 -> bus_creator/4  "BpedMove_No_Cnt"
  TCMode/1 -> bus_creator/5  "TCMode"
  ChimeBrk_B_Rq/1 -> bus_creator/6  "ChimeBrk_B_Rq"
  BrkLamp_B_Rq/1 -> bus_creator/7  "BrkLamp_B_Rq"
  DrvHdcLampInfo_D_Rq/1 -> bus_creator/8  "DrvHdcLampInfo_D_Rq"
  DrvHdcMsg_D_Rq/1 -> bus_creator/9  "DrvHdcMsg_D_Rq"
  HdcMde_D_Actl/1 -> bus_creator/10  "HdcMde_D_Actl"
  BrkBstrVac_B_Rq/1 -> bus_creator/11  "BrkBstrVac_B_Rq"
  TRLR_SWAY_CONFIG_STAT/1 -> bus_creator/12  "TRLR_SWAY_CONFIG_STAT"
  TRLR_SWAY_EVNT_IN_PROG/1 -> bus_creator/13  "TRLR_SWAY_EVNT_IN_PROG"
  DrvHdcWarnInfo_D_Rq/1 -> bus_creator/14  "DrvHdcWarnInfo_D_Rq"
  HsaMde_D_Mem/1 -> bus_creator/15  "HsaMde_D_Mem"
  HILL_DESC_MC/1 -> bus_creator/16  "HILL_DESC_MC"
  DrvSlipCtlMde_D_Ind/1 -> bus_creator/17  "DrvSlipCtlMde_D_Ind"
  DrvSlipCtlLamp_D_Rq/1 -> bus_creator/18  "DrvSlipCtlLamp_D_Rq"
  RearDiffElckrOpen_B_Rq/1 -> bus_creator/19  "RearDiffElckrOpen_B_Rq"
  DrvAntiLckLamp_D_Rq/1 -> bus_creator/20  "DrvAntiLckLamp_D_Rq"
  RearDiffLck_Tq2_RqMx/1 -> bus_creator/21  "RearDiffLck_Tq2_RqMx"

== system P702_NI_SoftECU/Output/Subsystem2/CAN_Signal/ABS_ESC/BrakeSysFeatures_3_0x41E ==
  ApaBrk_D_Stat : Constant  Value=0
  AutoHoldMde_D_Ind : Constant  Value=0
  AutoHoldMsgTxt_D_Rq : Constant  Value=0
  AutoHoldSwMde_B_Ind : Constant  Value=0
  BrkBstrVac_D_Stat : Constant  Value=0
  BrkMdeInhbt_B_RqDsply : Constant  Value=0
  CtaBrk_D_Stat : Constant  Value=0
  DrvSlipCtlMdeMsg_D_Rq : Constant  Value=0
  DrvSlipCtlOffLamp_D_Rq : Constant  Value=0
  RbaBrk_D_Stat : Constant  Value=0
  SelDrvMdeAwd_D_Rq : Constant  Value=0
  SelDrvMdeChassis2_D_Rq : Constant  Value=0
  SelDrvMdeChassis_D_Rq : Constant  Value=0
  TrailCtlMsgTxt_D_Rq : Constant  Value=0
  TrailCtl_D_Stat : Constant  Value=0
  bus_creator : BusCreator  Inputs=15
  out_port : Outport
  wires:
  bus_creator/1 -> out_port/1  "Subsystem2"
  AutoHoldMsgTxt_D_Rq/1 -> bus_creator/1  "AutoHoldMsgTxt_D_Rq"
  AutoHoldSwMde_B_Ind/1 -> bus_creator/2  "AutoHoldSwMde_B_Ind"
  AutoHoldMde_D_Ind/1 -> bus_creator/3  "AutoHoldMde_D_Ind"
  DrvSlipCtlMdeMsg_D_Rq/1 -> bus_creator/4  "DrvSlipCtlMdeMsg_D_Rq"
  BrkMdeInhbt_B_RqDsply/1 -> bus_creator/5  "BrkMdeInhbt_B_RqDsply"
  DrvSlipCtlOffLamp_D_Rq/1 -> bus_creator/6  "DrvSlipCtlOffLamp_D_Rq"
  BrkBstrVac_D_Stat/1 -> bus_creator/7  "BrkBstrVac_D_Stat"
  SelDrvMdeAwd_D_Rq/1 -> bus_creator/8  "SelDrvMdeAwd_D_Rq"
  SelDrvMdeChassis_D_Rq/1 -> bus_creator/9  "SelDrvMdeChassis_D_Rq"
  ApaBrk_D_Stat/1 -> bus_creator/10  "ApaBrk_D_Stat"
  CtaBrk_D_Stat/1 -> bus_creator/11  "CtaBrk_D_Stat"
  SelDrvMdeChassis2_D_Rq/1 -> bus_creator/12  "SelDrvMdeChassis2_D_Rq"
  TrailCtl_D_Stat/1 -> bus_creator/13  "TrailCtl_D_Stat"
  TrailCtlMsgTxt_D_Rq/1 -> bus_creator/14  "TrailCtlMsgTxt_D_Rq"
  RbaBrk_D_Stat/1 -> bus_creator/15  "RbaBrk_D_Stat"

== system P702_NI_SoftECU/Output/Subsystem2/CAN_Signal/ABS_ESC/DesiredTorqBrk_0x213 ==
  AbsActv_B_Actl : Constant  Value=0
  AccBrkActv_B_Actl : Constant  Value=0
  AccBrkDeny_B_Actl : Constant  Value=0
  AccBrkDis_B_Actl : Constant  Value=0
  AccBrkPrchgActv_B_Actl : Constant  Value=0
  AccBrkTotTqMn_B_Actl : Constant  Value=0
  AccBrkWarm_B_Actl : Constant  Value=0
  AccDis_B_ActlEpb : Constant  Value=0
  AccStopActv_B_ActlBrk : Constant  Value=0
  CcDis_B_Cmd : Constant  Value=0
  CmbbBaSensInc_B_Actl : Constant  Value=0
  CmbbBrkDecel_B_Actl : Constant  Value=0
  CmbbBrkDis_B_Actl : Constant  Value=0
  CmbbBrkPrchg_B_Actl : Constant  Value=0
  CmbbDeny_B_ActlBrk : Constant  Value=0
  LscmbBrkPrchg_B_Actl : Constant  Value=0
  LscmbbBaSensInc_B_Actl : Constant  Value=0
  LscmbbBrkDecel_B_Actl : Constant  Value=0
  LscmbbBrkDis_B_Actl : Constant  Value=0
  LscmbbDeny_B_ActlBrk : Constant  Value=0
  LscmbbMntr_B_Err : Constant  Value=0
  PrkBrkMsgTxt_D_Rq : Constant  Value=0
  PrkBrkRedLamp_D_Rq : Constant  Value=0
  PrkBrkStatus : Constant  Value=0
  PrkBrkYwLamp_D_Rq : Constant  Value=0
  PrplDrgCtlActv_B_Actl : Constant  Value=0
  PrplWhlTot_Tq_RqMx : Constant  Value=0
  StabCtlBrkActv_B_Actl : Constant  Value=0
  TracCtlPtActv_B_Actl : Constant  Value=0
  VehLongOvrGnd_A_Est : Constant  Value=0
  VehStop_D_Stat : Constant  Value=0
  VehicleStationary : Constant  Value=0
  bus_creator : BusCreator  Inputs=32
  out_port : Outport
  wires:
  bus_creator/1 -> out_port/1  "Subsystem2"
  PrplWhlTot_Tq_RqMx/1 -> bus_creator/1  "PrplWhlTot_Tq_RqMx"
  StabCtlBrkActv_B_Actl/1 -> bus_creator/2  "StabCtlBrkActv_B_Actl"
  AccStopActv_B_ActlBrk/1 -> bus_creator/3  "AccStopActv_B_ActlBrk"
  LscmbbBaSensInc_B_Actl/1 -> bus_creator/4  "LscmbbBaSensInc_B_Actl"
  LscmbbBrkDecel_B_Actl/1 -> bus_creator/5  "LscmbbBrkDecel_B_Actl"
  LscmbbBrkDis_B_Actl/1 -> bus_creator/6  "LscmbbBrkDis_B_Actl"
  LscmbbDeny_B_ActlBrk/1 -> bus_creator/7  "LscmbbDeny_B_ActlBrk"
  LscmbbMntr_B_Err/1 -> bus_creator/8  "LscmbbMntr_B_Err"
  LscmbBrkPrchg_B_Actl/1 -> bus_creator/9  "LscmbBrkPrchg_B_Actl"
  TracCtlPtActv_B_Actl/1 -> bus_creator/10  "TracCtlPtActv_B_Actl"
  PrkBrkRedLamp_D_Rq/1 -> bus_creator/11  "PrkBrkRedLamp_D_Rq"
  VehStop_D_Stat/1 -> bus_creator/12  "VehStop_D_Stat"
  PrkBrkStatus/1 -> bus_creator/13  "PrkBrkStatus"
  VehicleStationary/1 -> bus_creator/14  "VehicleStationary"
  PrkBrkYwLamp_D_Rq/1 -> bus_creator/15  "PrkBrkYwLamp_D_Rq"
  PrkBrkMsgTxt_D_Rq/1 -> bus_creator/16  "PrkBrkMsgTxt_D_Rq"
  AccDis_B_ActlEpb/1 -> bus_creator/17  "AccDis_B_ActlEpb"
  CcDis_B_Cmd/1 -> bus_creator/18  "CcDis_B_Cmd"
  PrplDrgCtlActv_B_Actl/1 -> bus_creator/19  "PrplDrgCtlActv_B_Actl"
  AbsActv_B_Actl/1 -> bus_creator/20  "AbsActv_B_Actl"
  AccBrkDis_B_Actl/1 -> bus_creator/21  "AccBrkDis_B_Actl"
  AccBrkActv_B_Actl/1 -> bus_creator/22  "AccBrkActv_B_Actl"
  AccBrkDeny_B_Actl/1 -> bus_creator/23  "AccBrkDeny_B_Actl"
  VehLongOvrGnd_A_Est/1 -> bus_creator/24  "VehLongOvrGnd_A_Est"
  AccBrkWarm_B_Actl/1 -> bus_creator/25  "AccBrkWarm_B_Actl"
  AccBrkTotTqMn_B_Actl/1 -> bus_creator/26  "AccBrkTotTqMn_B_Actl"
  AccBrkPrchgActv_B_Actl/1 -> bus_creator/27  "AccBrkPrchgActv_B_Actl"
  CmbbDeny_B_ActlBrk/1 -> bus_creator/28  "CmbbDeny_B_ActlBrk"
  CmbbBrkPrchg_B_Actl/1 -> bus_creator/29  "CmbbBrkPrchg_B_Actl"
  CmbbBrkDecel_B_Actl/1 -> bus_creator/30  "CmbbBrkDecel_B_Actl"
  CmbbBaSensInc_B_Actl/1 -> bus_creator/31  "CmbbBaSensInc_B_Actl"
  CmbbBrkDis_B_Actl/1 -> bus_creator/32  "CmbbBrkDis_B_Actl"

== system P702_NI_SoftECU/Output/Subsystem2/CAN_Signal/ABS_ESC/DesiredTorqBrk_2_0x214 ==
  PrplWhlRear_Tq_RqMn : Constant  Value=0
  PrplWhlRear_Tq_RqMx : Constant  Value=0
  PrplWhlTot_Tq_RqMn : Constant  Value=0
  PrplWhlTqRqMn_No_Cnt : Constant  Value=0
  PrplWhlTqRqMn_No_Cs : Constant  Value=0
  RgenBrkDynoMde_B_Actl : Constant  Value=0
  RgenTqFalt_B_Actl : Constant  Value=0
  bus_creator : BusCreator  Inputs=7
  out_port : Outport
  wires:
  bus_creator/1 -> out_port/1  "Subsystem2"
  PrplWhlTot_Tq_RqMn/1 -> bus_creator/1  "PrplWhlTot_Tq_RqMn"
  PrplWhlRear_Tq_RqMx/1 -> bus_creator/2  "PrplWhlRear_Tq_RqMx"
  PrplWhlRear_Tq_RqMn/1 -> bus_creator/3  "PrplWhlRear_Tq_RqMn"
  PrplWhlTqRqMn_No_Cs/1 -> bus_creator/4  "PrplWhlTqRqMn_No_Cs"
  PrplWhlTqRqMn_No_Cnt/1 -> bus_creator/5  "PrplWhlTqRqMn_No_Cnt"
  RgenTqFalt_B_Actl/1 -> bus_creator/6  "RgenTqFalt_B_Actl"
  RgenBrkDynoMde_B_Actl/1 -> bus_creator/7  "RgenBrkDynoMde_B_Actl"

== system P702_NI_SoftECU/Output/Subsystem2/CAN_Signal/ABS_ESC/Global_PATS_SubTarget_0x49 ==
  bus_creator : BusCreator  Inputs=2
  immoSubTarget1Cmd_T1 : Constant  Value=0
  immoSubTarget1Data_T1 : Constant  Value=0
  out_port : Outport
  wires:
  bus_creator/1 -> out_port/1  "Subsystem2"
  immoSubTarget1Cmd_T1/1 -> bus_creator/1  "immoSubTarget1Cmd_T1"
  immoSubTarget1Data_T1/1 -> bus_creator/2  "immoSubTarget1Data_T1"

== system P702_NI_SoftECU/Output/Subsystem2/CAN_Signal/ABS_ESC/SelectDriveModeData2_0x44E ==
  SelDrvMdePos01_D_Stat : Constant  Value=0
  SelDrvMdePos02_D_Stat : Constant  Value=0
  SelDrvMdePos03_D_Stat : Constant  Value=0
  SelDrvMdePos04_D_Stat : Constant  Value=0
  SelDrvMdePos05_D_Stat : Constant  Value=0
  SelDrvMdePos06_D_Stat : Constant  Value=0
  SelDrvMdePos07_D_Stat : Constant  Value=0
  SelDrvMdePos08_D_Stat : Constant  Value=0
  SelDrvMdePos09_D_Stat : Constant  Value=0
  SelDrvMdePos10_D_Stat : Constant  Value=0
  SelDrvMdePos11_D_Stat : Constant  Value=0
  SelDrvMdePos12_D_Stat : Constant  Value=0
  bus_creator : BusCreator  Inputs=12
  out_port : Outport
  wires:
  bus_creator/1 -> out_port/1  "Subsystem2"
  SelDrvMdePos01_D_Stat/1 -> bus_creator/1  "SelDrvMdePos01_D_Stat"
  SelDrvMdePos02_D_Stat/1 -> bus_creator/2  "SelDrvMdePos02_D_Stat"
  SelDrvMdePos03_D_Stat/1 -> bus_creator/3  "SelDrvMdePos03_D_Stat"
  SelDrvMdePos04_D_Stat/1 -> bus_creator/4  "SelDrvMdePos04_D_Stat"
  SelDrvMdePos05_D_Stat/1 -> bus_creator/5  "SelDrvMdePos05_D_Stat"
  SelDrvMdePos06_D_Stat/1 -> bus_creator/6  "SelDrvMdePos06_D_Stat"
  SelDrvMdePos07_D_Stat/1 -> bus_creator/7  "SelDrvMdePos07_D_Stat"
  SelDrvMdePos12_D_Stat/1 -> bus_creator/8  "SelDrvMdePos12_D_Stat"
  SelDrvMdePos11_D_Stat/1 -> bus_creator/9  "SelDrvMdePos11_D_Stat"
  SelDrvMdePos10_D_Stat/1 -> bus_creator/10  "SelDrvMdePos10_D_Stat"
  SelDrvMdePos09_D_Stat/1 -> bus_creator/11  "SelDrvMdePos09_D_Stat"
  SelDrvMdePos08_D_Stat/1 -> bus_creator/12  "SelDrvMdePos08_D_Stat"

== system P702_NI_SoftECU/Output/Subsystem2/CAN_Signal/ABS_ESC/SelectDriveModeData_0x420 ==
  ActvDrvMde_D2_Stat : Constant  Value=0
  AwdMde_D_RqBrk : Constant  Value=0
  SelDrvMdeMsgTxt_D_Rq : Constant  Value=0
  SelDrvMdePos01_B_Avail : Constant  Value=0
  SelDrvMdePos02_B_Avail : Constant  Value=0
  SelDrvMdePos03_B_Avail : Constant  Value=0
  SelDrvMdePos04_B_Avail : Constant  Value=0
  SelDrvMdePos05_B_Avail : Constant  Value=0
  SelDrvMdePos06_B_Avail : Constant  Value=0
  SelDrvMdePos07_B_Avail : Constant  Value=0
  SelDrvMdePos08_B_Avail : Constant  Value=0
  SelDrvMdePos09_B_Avail : Constant  Value=0
  SelDrvMdePos10_B_Avail : Constant  Value=0
  SelDrvMdePos11_B_Avail : Constant  Value=0
  SelDrvMdePos12_B_Avail : Constant  Value=0
  SelDrvMdePt_D_Rq : Constant  Value=0
  SelDrvMde_D2_Rq : Constant  Value=0
  SelDrvMde_D_Stat : Constant  Value=0
  bus_creator : BusCreator  Inputs=18
  out_port : Outport
  wires:
  bus_creator/1 -> out_port/1  "Subsystem2"
  SelDrvMdeMsgTxt_D_Rq/1 -> bus_creator/1  "SelDrvMdeMsgTxt_D_Rq"
  SelDrvMdePt_D_Rq/1 -> bus_creator/2  "SelDrvMdePt_D_Rq"
  SelDrvMde_D_Stat/1 -> bus_creator/3  "SelDrvMde_D_Stat"
  SelDrvMdePos01_B_Avail/1 -> bus_creator/4  "SelDrvMdePos01_B_Avail"
  AwdMde_D_RqBrk/1 -> bus_creator/5  "AwdMde_D_RqBrk"
  SelDrvMdePos02_B_Avail/1 -> bus_creator/6  "SelDrvMdePos02_B_Avail"
  SelDrvMdePos03_B_Avail/1 -> bus_creator/7  "SelDrvMdePos03_B_Avail"
  SelDrvMdePos04_B_Avail/1 -> bus_creator/8  "SelDrvMdePos04_B_Avail"
  SelDrvMdePos05_B_Avail/1 -> bus_creator/9  "SelDrvMdePos05_B_Avail"
  SelDrvMdePos06_B_Avail/1 -> bus_creator/10  "SelDrvMdePos06_B_Avail"
  SelDrvMdePos07_B_Avail/1 -> bus_creator/11  "SelDrvMdePos07_B_Avail"
  SelDrvMdePos08_B_Avail/1 -> bus_creator/12  "SelDrvMdePos08_B_Avail"
  SelDrvMdePos09_B_Avail/1 -> bus_creator/13  "SelDrvMdePos09_B_Avail"
  SelDrvMdePos10_B_Avail/1 -> bus_creator/14  "SelDrvMdePos10_B_Avail"
  SelDrvMdePos11_B_Avail/1 -> bus_creator/15  "SelDrvMdePos11_B_Avail"
  SelDrvMdePos12_B_Avail/1 -> bus_creator/16  "SelDrvMdePos12_B_Avail"
  ActvDrvMde_D2_Stat/1 -> bus_creator/17  "ActvDrvMde_D2_Stat"
  SelDrvMde_D2_Rq/1 -> bus_creator/18  "SelDrvMde_D2_Rq"

== system P702_NI_SoftECU/Output/Subsystem2/CAN_Signal/ABS_ESC/SteeringPinion_Data2_0x7F ==
  AwdLatDelta_B_Rq : Constant  Value=0
  AwdLatDelta_Tq_Rq : Constant  Value=0
  bus_creator : BusCreator  Inputs=2
  out_port : Outport
  wires:
  bus_creator/1 -> out_port/1  "Subsystem2"
  AwdLatDelta_B_Rq/1 -> bus_creator/1  "AwdLatDelta_B_Rq"
  AwdLatDelta_Tq_Rq/1 -> bus_creator/2  "AwdLatDelta_Tq_Rq"

== system P702_NI_SoftECU/Output/Subsystem2/CAN_Signal/ABS_ESC/TesterPhysicalResABS_0x768 ==
  TesterPhysicalResABS : Constant  Value=0
  bus_creator : BusCreator  Inputs=1
  out_port : Outport
  wires:
  bus_creator/1 -> out_port/1  "Subsystem2"
  TesterPhysicalResABS/1 -> bus_creator/1  "TesterPhysicalResABS"

== system P702_NI_SoftECU/Output/Subsystem2/CAN_Signal/ABS_ESC/TrailerBrakeData_0x412 ==
  TrlrBrk_Pc_Rq : Constant  Value=0
  VehPtch_An_Dsply : Constant  Value=0
  VehRol_An_Dsply : Constant  Value=0
  bus_creator : BusCreator  Inputs=3
  out_port : Outport
  wires:
  bus_creator/1 -> out_port/1  "Subsystem2"
  TrlrBrk_Pc_Rq/1 -> bus_creator/1  "TrlrBrk_Pc_Rq"
  VehPtch_An_Dsply/1 -> bus_creator/2  "VehPtch_An_Dsply"
  VehRol_An_Dsply/1 -> bus_creator/3  "VehRol_An_Dsply"

== system P702_NI_SoftECU/Output/Subsystem2/CAN_Signal/ABS_ESC/WheelData_0x216 ==
  BrkObdData_No_Actl : Constant  Value=0
  BrkObdIndex_No_Actl : Constant  Value=0
  WhlDirFl_D_Actl : Constant  Value=0
  WhlDirFr_D_Actl : Constant  Value=0
  WhlDirRl_D_Actl : Constant  Value=0
  WhlDirRr_D_Actl : Constant  Value=0
  WhlRotatFl_No_Cnt : Constant  Value=0
  WhlRotatFr_No_Cnt : Constant  Value=0
  WhlRotatRl_No_Cnt : Constant  Value=0
  WhlRotatRr_No_Cnt : Constant  Value=0
  bus_creator : BusCreator  Inputs=10
  out_port : Outport
  wires:
  bus_creator/1 -> out_port/1  "Subsystem2"
  WhlRotatFr_No_Cnt/1 -> bus_creator/1  "WhlRotatFr_No_Cnt"
  WhlRotatFl_No_Cnt/1 -> bus_creator/2  "WhlRotatFl_No_Cnt"
  WhlRotatRr_No_Cnt/1 -> bus_creator/3  "WhlRotatRr_No_Cnt"
  WhlRotatRl_No_Cnt/1 -> bus_creator/4  "WhlRotatRl_No_Cnt"
  WhlDirRl_D_Actl/1 -> bus_creator/5  "WhlDirRl_D_Actl"
  WhlDirFr_D_Actl/1 -> bus_creator/6  "WhlDirFr_D_Actl"
  WhlDirFl_D_Actl/1 -> bus_creator/7  "WhlDirFl_D_Actl"
  WhlDirRr_D_Actl/1 -> bus_creator/8  "WhlDirRr_D_Actl"
  BrkObdIndex_No_Actl/1 -> bus_creator/9  "BrkObdIndex_No_Actl"
  BrkObdData_No_Actl/1 -> bus_creator/10  "BrkObdData_No_Actl"

== system P702_NI_SoftECU/Output/Subsystem2/CAN_Signal/ABS_ESC/WheelSpeed_0x217 ==
  WhlFl_W_Meas : Constant  Value=0
  WhlFr_W_Meas : Constant  Value=0
  WhlRl_W_Meas : Constant  Value=0
  WhlRr_W_Meas : Constant  Value=0
  bus_creator : BusCreator  Inputs=4
  out_port : Outport
  wires:
  bus_creator/1 -> out_port/1  "Subsystem2"
  WhlFl_W_Meas/1 -> bus_creator/1  "WhlFl_W_Meas"
  WhlFr_W_Meas/1 -> bus_creator/2  "WhlFr_W_Meas"
  WhlRl_W_Meas/1 -> bus_creator/3  "WhlRl_W_Meas"
  WhlRr_W_Meas/1 -> bus_creator/4  "WhlRr_W_Meas"

== system P702_NI_SoftECU/Output/Subsystem2/CAN_Signal/ADAS/ACCDATA ==
  AccBrkDecel_B_Rq : Constant  Value=0
  AccBrkPrchg_B_Rq : Constant  Value=0
  AccBrkTot_A_Rq : Constant  Value=0
  AccCancl_B_Rq : Constant  Value=0
  AccPrpl_A_Rq : Constant  Value=0
  AccPrpl_A_Rq1 : Constant  Value=0
  AccStopStat_B_Rq : Constant  Value=0
  CmbbEngTqMn_B_Rq : Constant  Value=0
  bus_creator : BusCreator  Inputs=8
  out_port : Outport
  wires:
  bus_creator/1 -> out_port/1  "Subsystem2"
  AccBrkPrchg_B_Rq/1 -> bus_creator/1  "AccBrkPrchg_B_Rq"
  AccBrkDecel_B_Rq/1 -> bus_creator/2  "AccBrkDecel_B_Rq"
  AccStopStat_B_Rq/1 -> bus_creator/3  "AccStopStat_B_Rq"
  AccBrkTot_A_Rq/1 -> bus_creator/4  "AccBrkTot_A_Rq"
  CmbbEngTqMn_B_Rq/1 -> bus_creator/5  "CmbbEngTqMn_B_Rq"
  AccCancl_B_Rq/1 -> bus_creator/6  "AccCancl_B_Rq"
  AccPrpl_A_Rq/1 -> bus_creator/7  "AccPrpl_A_Rq"
  AccPrpl_A_Rq1/1 -> bus_creator/8  "AccPrpl_A_Rq1"

== system P702_NI_SoftECU/Output/Subsystem2/CAN_Signal/ADAS/ACCDATA_2 ==
  CmbbBaSens_D_Rq : Constant  Value=0
  CmbbBrkDecel_A_Rq : Constant  Value=0
  CmbbBrkDecel_B_Rq : Constant  Value=0
  CmbbBrkPrchg_D_Rq : Constant  Value=0
  bus_creator : BusCreator  Inputs=4
  out_port : Outport
  wires:
  bus_creator/1 -> out_port/1  "Subsystem2"
  CmbbBrkPrchg_D_Rq/1 -> bus_creator/1  "CmbbBrkPrchg_D_Rq"
  CmbbBrkDecel_A_Rq/1 -> bus_creator/2  "CmbbBrkDecel_A_Rq"
  CmbbBaSens_D_Rq/1 -> bus_creator/3  "CmbbBaSens_D_Rq"
  CmbbBrkDecel_B_Rq/1 -> bus_creator/4  "CmbbBrkDecel_B_Rq"
